simulink model "model_reg"  (R2016a)
settings: Solver=ode4  StartTime=0.0  StopTime=10.0  FixedStep=0.001  RelTol=1e-3
values from neighbouring files (symbols this model uses):
  lin = 2    [all2.m]    (also in dane.m = 1; zad1.m = 10)
  Rn = 0.0185    [dane.m]    (also in obiekt.m; zad1.m)
libraries: simulink x3
settings Model: Creator=Maciek  LastModifiedBy=Maciek

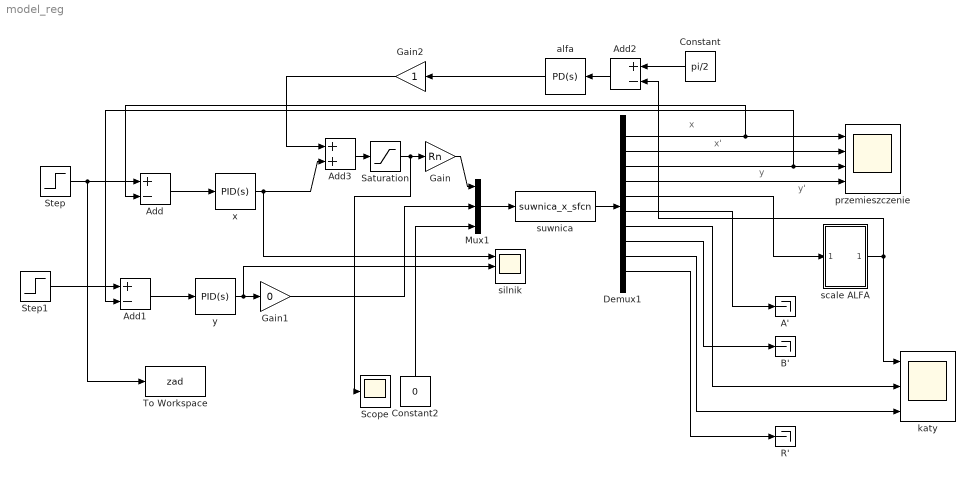
== system model_reg ==
  note: y'
  note: y
  note: x'
  note: x
  A' : Terminator
  Add : Sum  Inputs=+-
  Add1 : Sum  Inputs=+-
  Add2 : Sum  Inputs=+-
  Add3 : Sum
  B' : Terminator
  Constant : Constant  Value=pi/2
  Constant2 : Constant  Value=0
  Demux1 : Demux  Outputs=10
  Gain : Gain  Gain=Rn
  Gain1 : Gain  Gain=0
  Gain2 : Gain
  Mux1 : Mux  Inputs=3
  R' : Terminator
  Saturation : Saturate  UpperLimit=20  LowerLimit=-20
  Scope : Scope
  Step : Step  After=0.2  SampleTime=0
  Step1 : Step  After=0  SampleTime=0
  To Workspace : ToWorkspace  VariableName=zad  SaveFormat=Timeseries  SampleTime=-1
  alfa : simulink/Continuous/PID Controller  Controller=PD  TimeDomain=Continuous-time  SampleTime=-1  IntegratorMethod=Forward Euler  FilterMethod=Forward Euler  Form=Parallel  UseFilter=on  ControllerParametersSource=internal  P=220  I=0.015  D=5  N=100  InitialConditionSource=internal  InitialConditionForIntegrator=0  InitialConditionForFilter=0  ExternalReset=none  LimitOutput=on  UpperSaturationLimit=20  LowerSaturationLimit=-20  LinearizeAsGain=on  AntiWindupMode=none  Kb=1  TrackingMode=off  Kt=1  PParamMin=[]  PParamMax=[]  IParamMin=[]  IParamMax=[]  DParamMin=[]  DParamMax=[]  NParamMin=[]  NParamMax=[]  KbParamMin=[]  KbParamMax=[]  KtParamMin=[]  KtParamMax=[]  POutMin=[]  POutMax=[]  IOutMin=[]  IOutMax=[]  DOutMin=[]  DOutMax=[]  NOutMin=[]  NOutMax=[]  KbOutMin=[]  KbOutMax=[]  KtOutMin=[]  KtOutMax=[]  IntegratorOutMin=[]  IntegratorOutMax=[]  FilterOutMin=[]  FilterOutMax=[]  SumOutMin=[]  SumOutMax=[]  SumI1OutMin=[]  SumI1OutMax=[]  SumI2OutMin=[]  SumI2OutMax=[]  SumI3OutMin=[]  SumI3OutMax=[]  SumDOutMin=[]  SumDOutMax=[]  SaturationOutMin=[]  SaturationOutMax=[]  IntegratorContinuousStateAttributes=''  IntegratorStateMustResolveToSignalObject=off  IntegratorRTWStateStorageClass=Auto  FilterContinuousStateAttributes=''  FilterStateMustResolveToSignalObject=off  FilterRTWStateStorageClass=Auto  DifferentiatorICPrevScaledInput=0  DifferentiatorOutMin=[]  DifferentiatorOutMax=[]
  katy : Scope  NumInputPorts=3
  przemieszczenie : Scope  NumInputPorts=4
  scale ALFA : Subsystem
  silnik : Scope  NumInputPorts=3
  suwnica : S-Function  FunctionName=suwnica_x_sfcn  Parameters=x0  SFunctionDeploymentMode=off  EnableBusSupport=off
  x : simulink/Continuous/PID Controller  Controller=PID  TimeDomain=Continuous-time  SampleTime=-1  IntegratorMethod=Forward Euler  FilterMethod=Forward Euler  Form=Parallel  UseFilter=on  ControllerParametersSource=internal  P=220  I=0.005  D=2  N=100  InitialConditionSource=internal  InitialConditionForIntegrator=0  InitialConditionForFilter=0  ExternalReset=none  LimitOutput=on  UpperSaturationLimit=20  LowerSaturationLimit=-20  LinearizeAsGain=on  AntiWindupMode=none  Kb=1  TrackingMode=off  Kt=1  PParamMin=[]  PParamMax=[]  IParamMin=[]  IParamMax=[]  DParamMin=[]  DParamMax=[]  NParamMin=[]  NParamMax=[]  KbParamMin=[]  KbParamMax=[]  KtParamMin=[]  KtParamMax=[]  POutMin=[]  POutMax=[]  IOutMin=[]  IOutMax=[]  DOutMin=[]  DOutMax=[]  NOutMin=[]  NOutMax=[]  KbOutMin=[]  KbOutMax=[]  KtOutMin=[]  KtOutMax=[]  IntegratorOutMin=[]  IntegratorOutMax=[]  FilterOutMin=[]  FilterOutMax=[]  SumOutMin=[]  SumOutMax=[]  SumI1OutMin=[]  SumI1OutMax=[]  SumI2OutMin=[]  SumI2OutMax=[]  SumI3OutMin=[]  SumI3OutMax=[]  SumDOutMin=[]  SumDOutMax=[]  SaturationOutMin=[]  SaturationOutMax=[]  IntegratorContinuousStateAttributes=''  IntegratorStateMustResolveToSignalObject=off  IntegratorRTWStateStorageClass=Auto  FilterContinuousStateAttributes=''  FilterStateMustResolveToSignalObject=off  FilterRTWStateStorageClass=Auto  DifferentiatorICPrevScaledInput=0  DifferentiatorOutMin=[]  DifferentiatorOutMax=[]
  y : simulink/Continuous/PID Controller  Controller=PID  TimeDomain=Continuous-time  SampleTime=-1  IntegratorMethod=Forward Euler  FilterMethod=Forward Euler  Form=Parallel  UseFilter=on  ControllerParametersSource=internal  P=250  I=0.002  D=1  N=100  InitialConditionSource=internal  InitialConditionForIntegrator=0  InitialConditionForFilter=0  ExternalReset=none  LimitOutput=on  UpperSaturationLimit=20  LowerSaturationLimit=-20  LinearizeAsGain=on  AntiWindupMode=none  Kb=1  TrackingMode=off  Kt=1  PParamMin=[]  PParamMax=[]  IParamMin=[]  IParamMax=[]  DParamMin=[]  DParamMax=[]  NParamMin=[]  NParamMax=[]  KbParamMin=[]  KbParamMax=[]  KtParamMin=[]  KtParamMax=[]  POutMin=[]  POutMax=[]  IOutMin=[]  IOutMax=[]  DOutMin=[]  DOutMax=[]  NOutMin=[]  NOutMax=[]  KbOutMin=[]  KbOutMax=[]  KtOutMin=[]  KtOutMax=[]  IntegratorOutMin=[]  IntegratorOutMax=[]  FilterOutMin=[]  FilterOutMax=[]  SumOutMin=[]  SumOutMax=[]  SumI1OutMin=[]  SumI1OutMax=[]  SumI2OutMin=[]  SumI2OutMax=[]  SumI3OutMin=[]  SumI3OutMax=[]  SumDOutMin=[]  SumDOutMax=[]  SaturationOutMin=[]  SaturationOutMax=[]  IntegratorContinuousStateAttributes=''  IntegratorStateMustResolveToSignalObject=off  IntegratorRTWStateStorageClass=Auto  FilterContinuousStateAttributes=''  FilterStateMustResolveToSignalObject=off  FilterRTWStateStorageClass=Auto  DifferentiatorICPrevScaledInput=0  DifferentiatorOutMin=[]  DifferentiatorOutMax=[]
  wires:
  Mux1/1 -> suwnica/1
  Constant2/1 -> Mux1/3
  Demux1/10 -> R'/1
  Demux1/8 -> B'/1
  Demux1/7 -> katy/2
  Demux1/9 -> katy/3
  Demux1/6 -> A'/1
  Demux1/2 -> przemieszczenie/2
  Demux1/4 -> przemieszczenie/4
  suwnica/1 -> Demux1/1
  Demux1/5 -> scale ALFA/1(In1)
  Demux1/1 -> Add/2, przemieszczenie/1
  scale ALFA/1(Out1) -> Add2/2, katy/1
  Add/1 -> x/1
  Step/1 -> To Workspace/1, Add/1
  y/1 -> silnik/2, Gain1/1
  Demux1/3 -> Add1/2, przemieszczenie/3
  Add1/1 -> y/1
  Step1/1 -> Add1/1
  Gain1/1 -> Mux1/2
  Add2/1 -> alfa/1
  Constant/1 -> Add2/1
  alfa/1 -> Gain2/1
  Add3/1 -> Saturation/1
  x/1 -> Add3/2, silnik/1
  Saturation/1 -> Scope/1, Gain/1
  Gain/1 -> Mux1/1
  Gain2/1 -> Add3/1

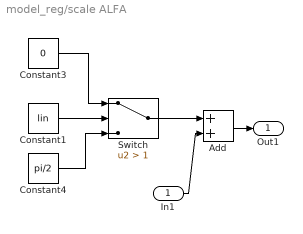
== system model_reg/scale ALFA ==
  In1 : Inport
  Add : Sum  Inputs=2
  Constant1 : Constant  Value=lin
  Constant3 : Constant  Value=0
  Constant4 : Constant  Value=pi/2
  Switch : Switch  Criteria=u2 > Threshold  Threshold=1
  Out1 : Outport
  wires:
  Add/1 -> Out1/1
  In1/1 -> Add/2
  Constant4/1 -> Switch/3
  Constant3/1 -> Switch/1
  Switch/1 -> Add/1
  Constant1/1 -> Switch/2
